simulink model "testing_posi_5"  (R2025a)
settings: Solver=ode4  StartTime=t_init  StopTime=t_end  FixedStep=t_step  RelTol=1e-3
undefined symbols (not defined in the file): L, loci, side, Twaitaddi, vi
settings Model: VariantFading=off  Creator=LEGION  LastModifiedBy=LEGION
settings ModelReferenceCC: EnableRefExpFcnMdlSchedulingChecks=on
settings RTWCC: GPUComputeCapability=3.5

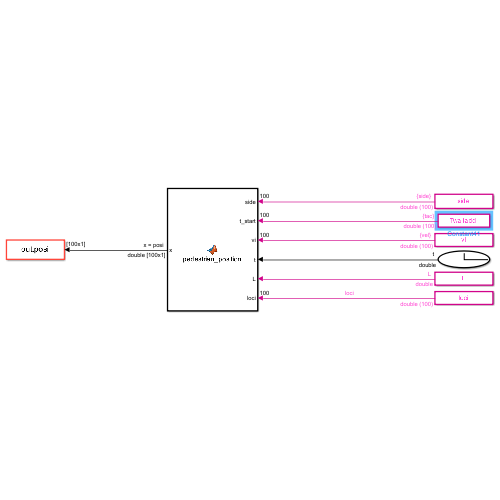
[thumbnail: Simulink's stored preview of the top-level diagram]
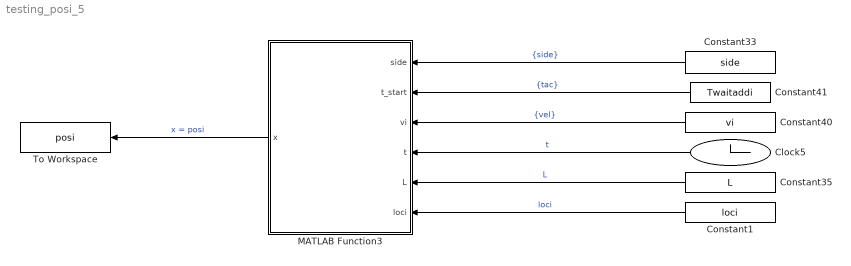
== system testing_posi_5 ==
  Clock5 : Clock
  Constant1 : Constant  Value=loci
  Constant33 : Constant  Value=side
  Constant35 : Constant  Value=L
  Constant40 : Constant  Value=vi
  Constant41 : Constant  Value=Twaitaddi
  MATLAB Function3 : MATLAB Function  TreatAsAtomicUnit=on
  To Workspace : ToWorkspace  VariableName=posi  SaveFormat=Timeseries  SampleTime=-1
  wires:
  Constant33/1 -> MATLAB Function3/1(side)  "{side}"
  Constant40/1 -> MATLAB Function3/3(vi)  "{vel}"
  Constant41/1 -> MATLAB Function3/2(t_start)  "{tac}"
  Constant35/1 -> MATLAB Function3/5(L)  "L"
  Clock5/1 -> MATLAB Function3/4(t)  "t"
  MATLAB Function3/1(x) -> To Workspace/1  "x = posi"
  Constant1/1 -> MATLAB Function3/6(loci)  "loci"

== matlab function testing_posi_5/MATLAB Function3 ==
  data: side input; x output; t_start input; vi input; t input; L input; loci input
function x = pedestrian_position(side, t_start, vi, t, L, loci)
% PEDESTRIAN_POSITION Determines the position of all pedestrians on the bridge.
%
% This function calculates the longitudinal position 'x' of pedestrians
% considering reflective boundaries (they turn around at 0 and L).
%
% INPUTS:
%   side    : Vector (Px1). Entry side (0: Left/Start, 1: Right/End).
%             Determines the initial walking direction.
%   t_start : Scalar. Time when the pedestrians start moving (s).
%   vi      : Vector (Px1). Walking speed (m/s).
%   t       : Scalar. Current simulation time (s).
%   L       : Scalar. Length of the bridge (m).
%   loci      : Vector (Px1). Initial position of pedestrians along the bridge (m).
%
% OUTPUTS:
%   x       : Vector (Px1). Current position of pedestrians (m).

    % 1. Determine Direction
    % Convert side (0 or 1) to a direction scalar (+1 or -1).
    % If side is 0 (Left), direction is +1. If side is 1 (Right), direction is -1.
    direction = 1 - 2 .* side; 

    % 2. Calculate Active Time
    % Calculate how long they have been walking. Result is 0 if t < t_start.
    delta_t = max(t - t_start, 0);

    % 3. Compute Virtual Position (Unbounded)
    % This is the position assuming the bridge is infinite.
    % Equation: x_virt = x_initial + (direction * speed * time)
    x_virtual = loci + (direction .* vi .* delta_t);

    % 4. Apply Reflective Boundaries (The "Folding" Logic)
    % We map the virtual position to a cycle of 2*L to simulate bouncing.
    cycle_pos = mod(x_virtual, 2*L);
    
    % Fold the domain to keep x within [0, L]
    x = min(cycle_pos, 2*L - cycle_pos);

    % 5. Handle Pre-Start State
    % Requirement: Before 't_start', pedestrians must be at x = 0.
    % If the current time t is less than t_start, force position to 0.
    if t < t_start
        x(:) = 0;
    end

end
